simulink model "CSDProj1Q1"  (R2019b)
settings: Solver=VariableStepAuto  StartTime=0.0  StopTime=250  RelTol=1e-3
values from neighbouring files (symbols this model uses):
  a_yr1_amp = 3    [CSDProj1Q1.m]
  a_yr1_time = 0    [CSDProj1Q1.m]
  a_yr2_amp = 3    [CSDProj1Q1.m]
  a_yr2_time = 0.01    [CSDProj1Q1.m]
  k_Theta = 1.5    [CSDProj1Q1.m]
  k_V_tilde = 10    [CSDProj1Q1.m]
  Ka = 4.3    [CSDProj1Q1.m]
  m = 1230    [CSDProj1Q1.m]    (also in CSDProj1Q2.m = 100)
  V0 = 40 * (1000/3600)    (= 11.1111111111)    [CSDProj1Q1.m]
  V_nom = 40 * (1000/3600)    (= 11.1111111111)    [CSDProj1Q1.m]
  Vw = 5    [CSDProj1Q1.m]
  w_ap = 3.2    [CSDProj1Q1.m]
  zeta_ap = 0.75    [CSDProj1Q1.m]
settings Model: Creator=shlomishetrit  LastModifiedBy=shlomishetrit

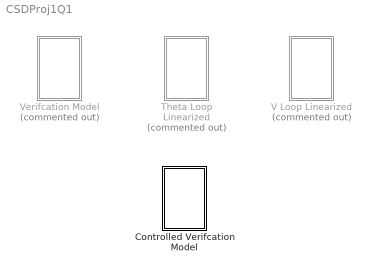
== system CSDProj1Q1 ==
  "Controlled Verifcation Model " : Subsystem
  Theta Loop Linearized : Subsystem  Commented=on
  V Loop Linearized : Subsystem  Commented=on
  "Verifcation Model " : Subsystem  Commented=on

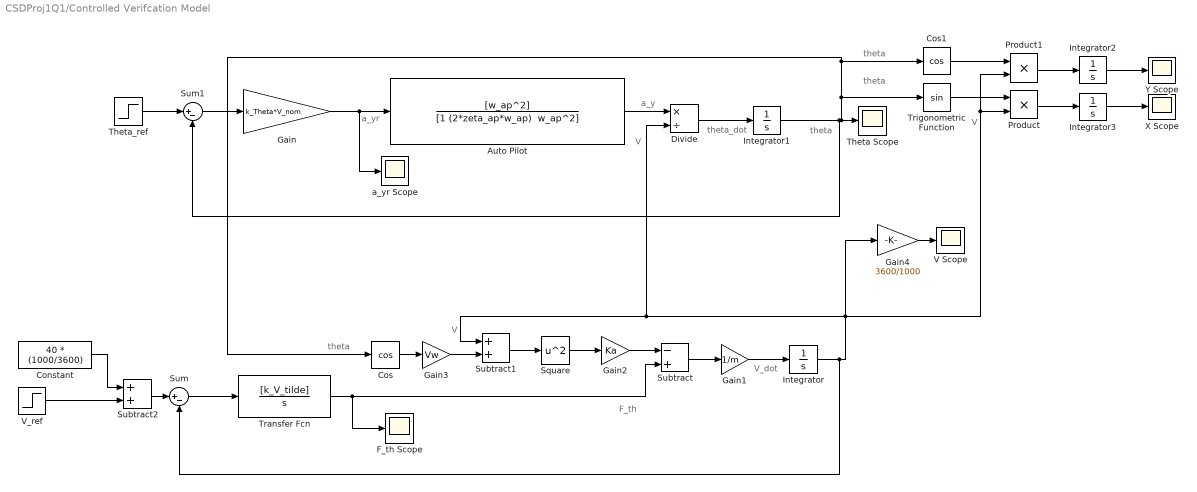
== system CSDProj1Q1/Controlled Verifcation Model  ==
  note: theta
  note: theta
  note: V
  note: V_dot
  note: theta
  note: theta
  note: theta_dot
  note: a_yr
  note: V
  note: F_th
  note: V
  note: a_y
  Auto Pilot : TransferFcn  Numerator=[w_ap^2]  Denominator="[1 (2*zeta_ap*w_ap)  w_ap^2]"  ContinuousStateAttributes='auto_pilot'
  Constant : Constant  Value=40 * (1000/3600)
  Cos : Trigonometry  Operator=cos
  Cos1 : Trigonometry  Operator=cos
  Divide : Product  Inputs=*/
  F_th Scope : Scope
  Gain : Gain  Gain=k_Theta*V_nom
  Gain1 : Gain  Gain=1/m
  Gain2 : Gain  Gain=Ka
  Gain3 : Gain  Gain=Vw
  Gain4 : Gain  Gain=3600/1000
  Integrator : Integrator  InitialCondition=V0
  Integrator1 : Integrator
  Integrator2 : Integrator
  Integrator3 : Integrator
  Product : Product
  Product1 : Product
  Square : Math  Operator=square  SignedPower=off  SaturateOnIntegerOverflow=on
  Subtract : Sum  Inputs=-+
  Subtract1 : Sum
  Subtract2 : Sum
  Sum : Sum  Inputs=|+-
  Sum1 : Sum  Inputs=|+-
  Theta Scope : Scope
  Theta_ref : Step  Time=50  After=deg2rad(180)  SampleTime=0
  Transfer Fcn : TransferFcn  Numerator=[k_V_tilde]  Denominator=[1 0]
  Trigonometric Function : Trigonometry
  V Scope : Scope
  V_ref : Step  Time=0  After=10 * (1000/3600)  SampleTime=0
  X Scope : Scope
  "Y Scope " : Scope
  a_yr Scope : Scope
  wires:
  Divide/1 -> Integrator1/1
  Sum1/1 -> Gain/1
  Transfer Fcn/1 -> Subtract/2, F_th Scope/1
  Integrator2/1 -> "Y Scope "/1
  Integrator/1 -> Gain4/1, Product/2, Product1/2, Subtract1/1, Divide/2, Sum/2
  Square/1 -> Gain2/1
  Gain2/1 -> Subtract/1
  Integrator1/1 -> Sum1/2, Theta Scope/1, Trigonometric Function/1, Cos/1, Cos1/1
  Auto Pilot/1 -> Divide/1
  Trigonometric Function/1 -> Product/1
  Gain3/1 -> Subtract1/2
  Cos/1 -> Gain3/1
  Product1/1 -> Integrator2/1
  Gain1/1 -> Integrator/1
  Integrator3/1 -> X Scope/1
  Subtract/1 -> Gain1/1
  Subtract1/1 -> Square/1
  Product/1 -> Integrator3/1
  Cos1/1 -> Product1/1
  Sum/1 -> Transfer Fcn/1
  Theta_ref/1 -> Sum1/1
  Gain/1 -> Auto Pilot/1, a_yr Scope/1
  Subtract2/1 -> Sum/1
  V_ref/1 -> Subtract2/2
  Constant/1 -> Subtract2/1
  Gain4/1 -> V Scope/1

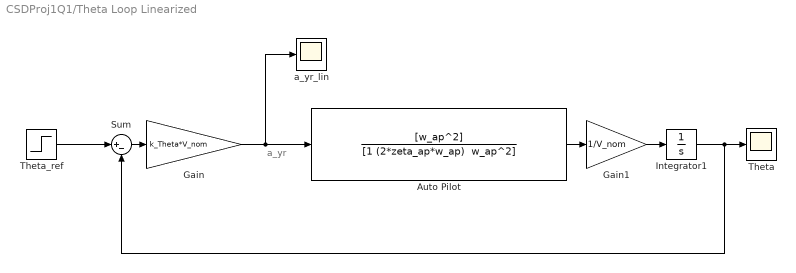
== system CSDProj1Q1/Theta Loop Linearized ==
  note: a_yr
  Auto Pilot : TransferFcn  Numerator=[w_ap^2]  Denominator="[1 (2*zeta_ap*w_ap)  w_ap^2]"  ContinuousStateAttributes='auto_pilot'
  Gain : Gain  Gain=k_Theta*V_nom
  Gain1 : Gain  Gain=1/V_nom
  Integrator1 : Integrator
  Sum : Sum  Inputs=|+-
  Theta : Scope
  Theta_ref : Step  Time=50  After=deg2rad(180)  SampleTime=0
  a_yr_lin : Scope
  wires:
  Gain/1 -> a_yr_lin/1, Auto Pilot/1
  Theta_ref/1 -> Sum/1
  Auto Pilot/1 -> Gain1/1
  Integrator1/1 -> Sum/2, Theta/1
  Sum/1 -> Gain/1
  Gain1/1 -> Integrator1/1

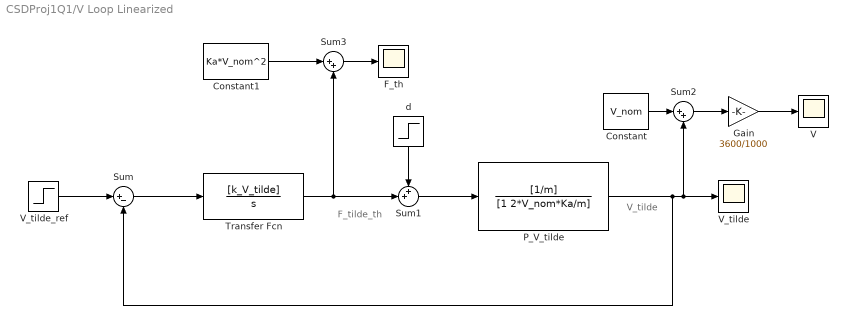
== system CSDProj1Q1/V Loop Linearized ==
  note: V_tilde
  note: F_tilde_th
  Constant : Constant  Value=V_nom
  Constant1 : Constant  Value=Ka*V_nom^2
  F_th : Scope
  Gain : Gain  Gain=3600/1000
  P_V_tilde : TransferFcn  Numerator=[1/m]  Denominator=[1 2*V_nom*Ka/m]  ContinuousStateAttributes='auto_pilot'
  Sum : Sum  Inputs=|+-
  Sum1 : Sum  Inputs=++|
  Sum2 : Sum  Inputs=|++
  Sum3 : Sum  Inputs=|++
  Transfer Fcn : TransferFcn  Numerator=[k_V_tilde]  Denominator=[1 0]
  V : Scope
  V_tilde : Scope
  V_tilde_ref : Step  Time=0  After=10 * (1000/3600)  SampleTime=0
  d : Step  Time=50  After=-1  SampleTime=0
  wires:
  Sum/1 -> Transfer Fcn/1
  P_V_tilde/1 -> Sum2/2, V_tilde/1, Sum/2
  V_tilde_ref/1 -> Sum/1
  Transfer Fcn/1 -> Sum3/2, Sum1/2
  Sum1/1 -> P_V_tilde/1
  d/1 -> Sum1/1
  Constant/1 -> Sum2/1
  Sum2/1 -> Gain/1
  Constant1/1 -> Sum3/1
  Sum3/1 -> F_th/1
  Gain/1 -> V/1

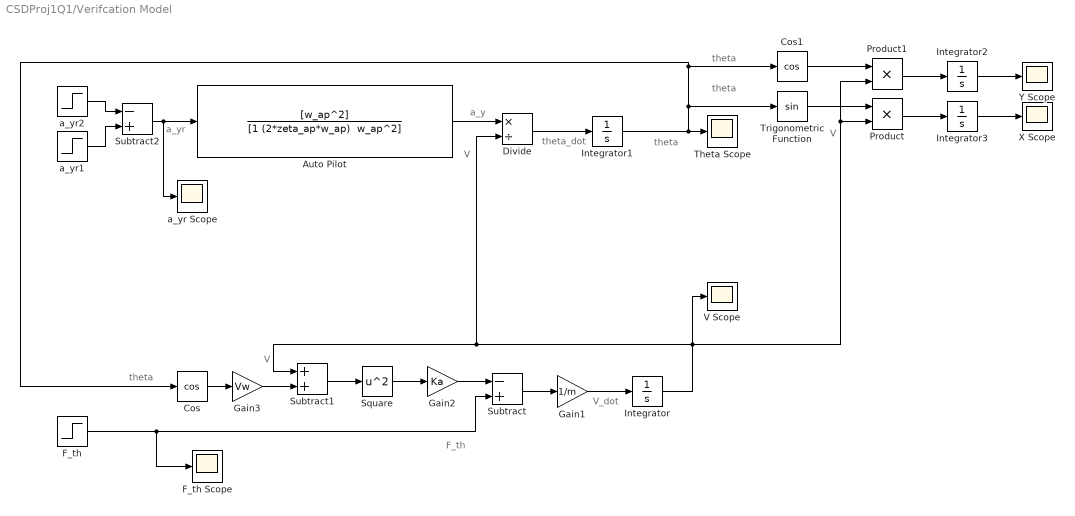
== system CSDProj1Q1/Verifcation Model  ==
  note: a_y
  note: V
  note: F_th
  note: V
  note: a_yr
  note: theta_dot
  note: theta
  note: theta
  note: V_dot
  note: V
  note: theta
  note: theta
  Auto Pilot : TransferFcn  Numerator=[w_ap^2]  Denominator="[1 (2*zeta_ap*w_ap)  w_ap^2]"  ContinuousStateAttributes='auto_pilot'
  Cos : Trigonometry  Operator=cos
  Cos1 : Trigonometry  Operator=cos
  Divide : Product  Inputs=*/
  F_th : Step  Time=0  After=1500  SampleTime=0
  F_th Scope : Scope
  Gain1 : Gain  Gain=1/m
  Gain2 : Gain  Gain=Ka
  Gain3 : Gain  Gain=Vw
  Integrator : Integrator  InitialCondition=V0
  Integrator1 : Integrator
  Integrator2 : Integrator
  Integrator3 : Integrator
  Product : Product
  Product1 : Product
  Square : Math  Operator=square  SignedPower=off  SaturateOnIntegerOverflow=on
  Subtract : Sum  Inputs=-+
  Subtract1 : Sum
  Subtract2 : Sum  Inputs=-+
  Theta Scope : Scope
  Trigonometric Function : Trigonometry
  V Scope : Scope
  X Scope : Scope
  "Y Scope " : Scope
  a_yr Scope : Scope
  a_yr1 : Step  Time=a_yr1_time  After=a_yr1_amp  SampleTime=0
  a_yr2 : Step  Time=a_yr2_time  After=a_yr2_amp  SampleTime=0
  wires:
  Cos1/1 -> Product1/1
  Product/1 -> Integrator3/1
  Subtract1/1 -> Square/1
  Subtract/1 -> Gain1/1
  Integrator3/1 -> X Scope/1
  Gain1/1 -> Integrator/1
  Product1/1 -> Integrator2/1
  Cos/1 -> Gain3/1
  Gain3/1 -> Subtract1/2
  a_yr2/1 -> Subtract2/1
  Trigonometric Function/1 -> Product/1
  Auto Pilot/1 -> Divide/1
  Integrator1/1 -> Cos1/1, Cos/1, Trigonometric Function/1, Theta Scope/1
  a_yr1/1 -> Subtract2/2
  Gain2/1 -> Subtract/1
  Square/1 -> Gain2/1
  Integrator/1 -> Divide/2, Subtract1/1, Product1/2, Product/2, V Scope/1
  Integrator2/1 -> "Y Scope "/1
  F_th/1 -> F_th Scope/1, Subtract/2
  Subtract2/1 -> a_yr Scope/1, Auto Pilot/1
  Divide/1 -> Integrator1/1
